simulink model "god"  (R2018a)
settings: Solver=VariableStepAuto  StartTime=0.0  StopTime=10  FixedStep=0.01  RelTol=1e-3
libraries: instrumentlib x14
settings Model: EnablePacing=on  Creator=U500304  LastModifiedBy=U500304
settings SolverCC: ZeroCrossAlgorithm=Adaptive
settings DataIOCC: SaveOutput=off  SaveTime=off
settings DebuggingCC: MaxConsecutiveZCsMsg=none

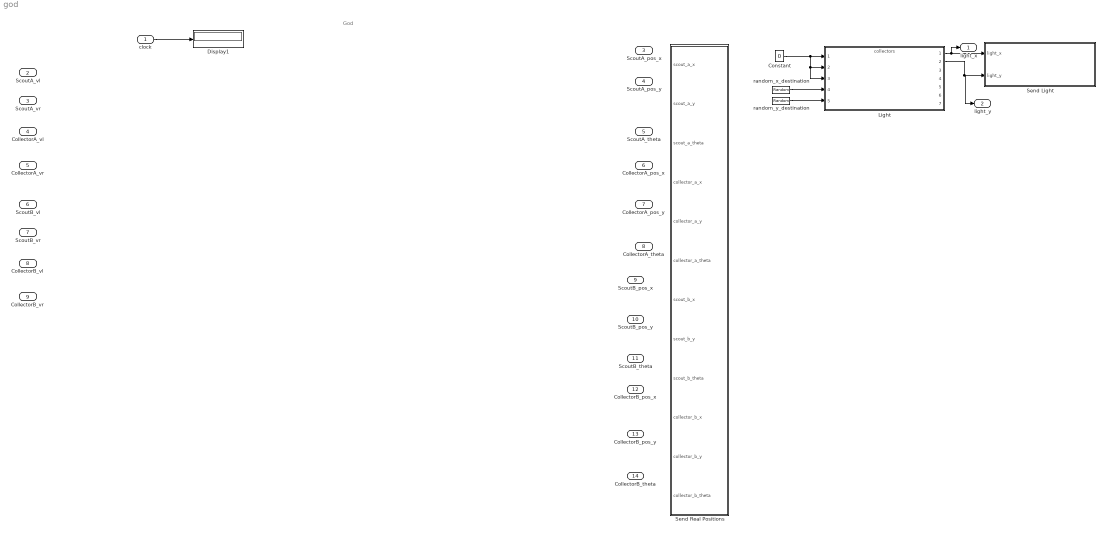
== system god ==
  note: God
  clock : Inport  OutDataTypeStr=double  PortDimensions=1  SampleTime=0
  ScoutA_vl : Inport  Port=2
  ScoutA_vr : Inport  Port=3
  CollectorA_vl : Inport  Port=4
  CollectorA_vr : Inport  Port=5
  ScoutB_vl : Inport  Port=6
  ScoutB_vr : Inport  Port=7
  CollectorB_vl : Inport  Port=8
  CollectorB_vr : Inport  Port=9
  Constant : Constant  Value=0
  Display1 : Display
  Light : ModelReference  ModelNameDialog=collectors  SimulationMode=Normal  ModelReferenceVersion=1.198
  Send Light : Subsystem
  Send Real Positions : Subsystem
  random_x_destination : UniformRandomNumber  Minimum=0  Maximum=199  Seed=14  SampleTime=1
  random_y_destination : UniformRandomNumber  Minimum=0  Maximum=99  Seed=66  SampleTime=1
  light_x : Outport
  light_y : Outport  Port=2
  ScoutA_pos_x : Outport  Port=3
  ScoutA_pos_y : Outport  Port=4
  ScoutA_theta : Outport  Port=5
  CollectorA_pos_x : Outport  Port=6
  CollectorA_pos_y : Outport  Port=7
  CollectorA_theta : Outport  Port=8
  ScoutB_pos_x : Outport  Port=9
  ScoutB_pos_y : Outport  Port=10
  ScoutB_theta : Outport  Port=11
  CollectorB_pos_x : Outport  Port=12
  CollectorB_pos_y : Outport  Port=13
  CollectorB_theta : Outport  Port=14
  wires:
  clock/1 -> Display1/1
  random_x_destination/1 -> Light/4
  random_y_destination/1 -> Light/5
  Constant/1 -> Light/3, Light/2, Light/1
  Light/1 -> light_x/1, Send Light/1(light_x)
  Light/2 -> light_y/1, Send Light/2(light_y)
  ? -> ScoutA_pos_x/1, Send Real Positions/1(scout_a_x)
  ? -> ScoutA_pos_y/1, Send Real Positions/2(scout_a_y)
  ? -> ScoutA_theta/1, Send Real Positions/3(scout_a_theta)
  ? -> CollectorA_pos_x/1, Send Real Positions/4(collector_a_x)
  ? -> CollectorA_pos_y/1, Send Real Positions/5(collector_a_y)
  ? -> CollectorA_theta/1, Send Real Positions/6(collector_a_theta)
  ? -> ScoutB_pos_x/1, Send Real Positions/7(scout_b_x)
  ? -> ScoutB_pos_y/1, Send Real Positions/8(scout_b_y)
  ? -> ScoutB_theta/1, Send Real Positions/9(scout_b_theta)
  ? -> CollectorB_pos_x/1, Send Real Positions/10(collector_b_x)
  ? -> CollectorB_pos_y/1, Send Real Positions/11(collector_b_y)
  ? -> CollectorB_theta/1, Send Real Positions/12(collector_b_theta)

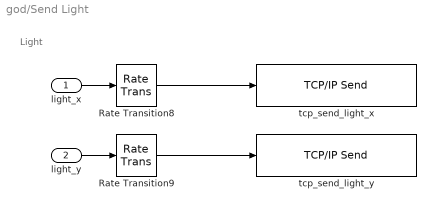
== system god/Send Light ==
  note: Light
  light_x : Inport
  light_y : Inport  Port=2
  Rate Transition8 : RateTransition  OutPortSampleTime=0.1
  Rate Transition9 : RateTransition  OutPortSampleTime=0.1
  tcp_send_light_x : instrumentlib/TCP//IP Send  Host=localhost  Port=50013  EnableBlockingMode=on  Timeout=1  ByteOrder=LittleEndian  TransferDelay=on
      settings: SourceProductName=Instrument Control Toolbox
  tcp_send_light_y : instrumentlib/TCP//IP Send  Host=localhost  Port=50014  EnableBlockingMode=on  Timeout=1  ByteOrder=LittleEndian  TransferDelay=on
      settings: SourceProductName=Instrument Control Toolbox
  wires:
  light_y/1 -> Rate Transition9/1
  light_x/1 -> Rate Transition8/1
  Rate Transition8/1 -> tcp_send_light_x/1
  Rate Transition9/1 -> tcp_send_light_y/1

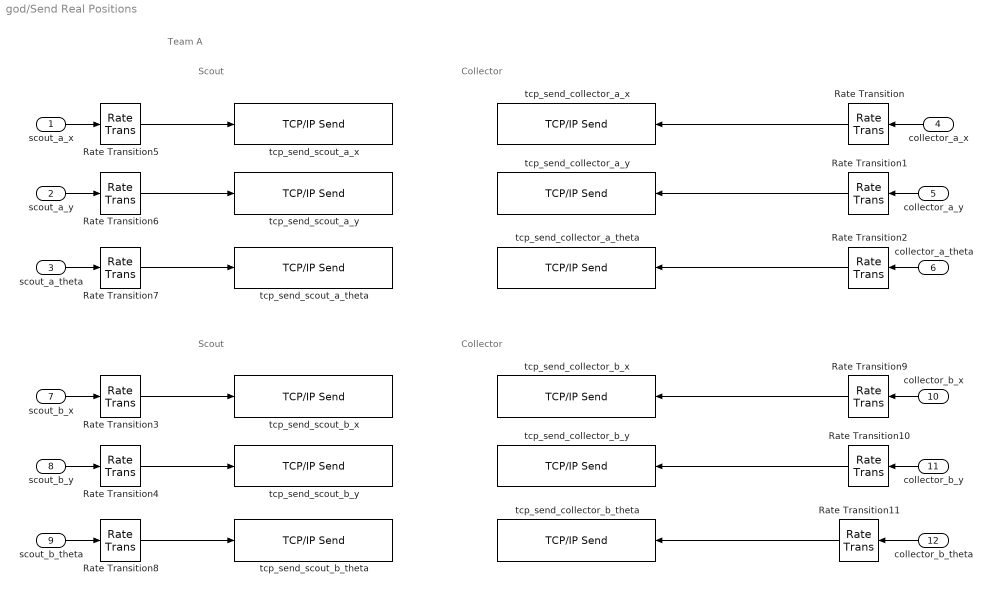
== system god/Send Real Positions ==
  note: Team A
  note: Scout
  note: Collector
  note: Scout
  note: Collector
  scout_a_x : Inport
  scout_a_y : Inport  Port=2
  scout_a_theta : Inport  Port=3
  collector_a_x : Inport  Port=4
  collector_a_y : Inport  Port=5
  collector_a_theta : Inport  Port=6
  scout_b_x : Inport  Port=7
  scout_b_y : Inport  Port=8
  scout_b_theta : Inport  Port=9
  collector_b_x : Inport  Port=10
  collector_b_y : Inport  Port=11
  collector_b_theta : Inport  Port=12
  Rate Transition{,1..11} (12 alike) : RateTransition  OutPortSampleTime=0.1
  tcp_send_collector_a_theta : instrumentlib/TCP//IP Send  Host=localhost  Port=50006  EnableBlockingMode=on  Timeout=1  ByteOrder=LittleEndian  TransferDelay=on
      settings: SourceProductName=Instrument Control Toolbox
  tcp_send_collector_a_x : instrumentlib/TCP//IP Send  Host=localhost  Port=50004  EnableBlockingMode=on  Timeout=1  ByteOrder=LittleEndian  TransferDelay=on
      settings: SourceProductName=Instrument Control Toolbox
  tcp_send_collector_a_y : instrumentlib/TCP//IP Send  Host=localhost  Port=50005  EnableBlockingMode=on  Timeout=1  ByteOrder=LittleEndian  TransferDelay=on
      settings: SourceProductName=Instrument Control Toolbox
  tcp_send_collector_b_theta : instrumentlib/TCP//IP Send  Host=localhost  Port=50012  EnableBlockingMode=on  Timeout=1  ByteOrder=LittleEndian  TransferDelay=on
      settings: SourceProductName=Instrument Control Toolbox
  tcp_send_collector_b_x : instrumentlib/TCP//IP Send  Host=localhost  Port=50010  EnableBlockingMode=on  Timeout=1  ByteOrder=LittleEndian  TransferDelay=on
      settings: SourceProductName=Instrument Control Toolbox
  tcp_send_collector_b_y : instrumentlib/TCP//IP Send  Host=localhost  Port=50011  EnableBlockingMode=on  Timeout=1  ByteOrder=LittleEndian  TransferDelay=on
      settings: SourceProductName=Instrument Control Toolbox
  tcp_send_scout_a_theta : instrumentlib/TCP//IP Send  Host=localhost  Port=50003  EnableBlockingMode=on  Timeout=1  ByteOrder=LittleEndian  TransferDelay=on
      settings: SourceProductName=Instrument Control Toolbox
  tcp_send_scout_a_x : instrumentlib/TCP//IP Send  Host=localhost  Port=50001  EnableBlockingMode=on  Timeout=1  ByteOrder=LittleEndian  TransferDelay=on
      settings: SourceProductName=Instrument Control Toolbox
  tcp_send_scout_a_y : instrumentlib/TCP//IP Send  Host=localhost  Port=50002  EnableBlockingMode=on  Timeout=1  ByteOrder=LittleEndian  TransferDelay=on
      settings: SourceProductName=Instrument Control Toolbox
  tcp_send_scout_b_theta : instrumentlib/TCP//IP Send  Host=localhost  Port=50009  EnableBlockingMode=on  Timeout=1  ByteOrder=LittleEndian  TransferDelay=on
      settings: SourceProductName=Instrument Control Toolbox
  tcp_send_scout_b_x : instrumentlib/TCP//IP Send  Host=localhost  Port=50007  EnableBlockingMode=on  Timeout=1  ByteOrder=LittleEndian  TransferDelay=on
      settings: SourceProductName=Instrument Control Toolbox
  tcp_send_scout_b_y : instrumentlib/TCP//IP Send  Host=localhost  Port=50008  EnableBlockingMode=on  Timeout=1  ByteOrder=LittleEndian  TransferDelay=on
      settings: SourceProductName=Instrument Control Toolbox
  wires:
  collector_b_x/1 -> Rate Transition9/1
  scout_a_x/1 -> Rate Transition5/1
  collector_b_y/1 -> Rate Transition10/1
  collector_a_x/1 -> Rate Transition/1
  scout_a_y/1 -> Rate Transition6/1
  collector_a_y/1 -> Rate Transition1/1
  collector_a_theta/1 -> Rate Transition2/1
  collector_b_theta/1 -> Rate Transition11/1
  scout_a_theta/1 -> Rate Transition7/1
  scout_b_theta/1 -> Rate Transition8/1
  scout_b_y/1 -> Rate Transition4/1
  scout_b_x/1 -> Rate Transition3/1
  Rate Transition/1 -> tcp_send_collector_a_x/1
  Rate Transition1/1 -> tcp_send_collector_a_y/1
  Rate Transition2/1 -> tcp_send_collector_a_theta/1
  Rate Transition5/1 -> tcp_send_scout_a_x/1
  Rate Transition6/1 -> tcp_send_scout_a_y/1
  Rate Transition7/1 -> tcp_send_scout_a_theta/1
  Rate Transition3/1 -> tcp_send_scout_b_x/1
  Rate Transition4/1 -> tcp_send_scout_b_y/1
  Rate Transition8/1 -> tcp_send_scout_b_theta/1
  Rate Transition9/1 -> tcp_send_collector_b_x/1
  Rate Transition10/1 -> tcp_send_collector_b_y/1
  Rate Transition11/1 -> tcp_send_collector_b_theta/1
